simulink subsystem "Propulsion"  (R2023b)
settings: Solver=VariableStepAuto  StartTime=0.0  StopTime=10.0  RelTol=1e-3
undefined symbols (not defined in the file): Thrust, Ts
settings Model: Creator=szdaniel  LastModifiedBy=szdaniel

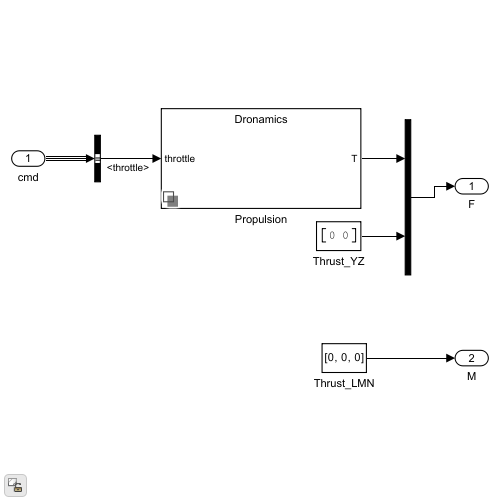
[thumbnail: Simulink's stored preview of the top-level diagram]
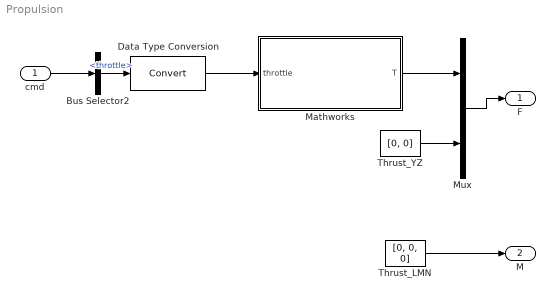
== system Propulsion ==
  cmd : Inport  OutDataTypeStr=Bus: PilotCmdBus  SampleTime=Ts
  Bus Selector2 : BusSelector  OutputSignals=throttle
  Data Type Conversion : DataTypeConversion  SaturateOnIntegerOverflow=off  RndMeth=Floor
  Mathworks : Subsystem  VariantControl=LowFidelityPropulsion
  Mux : Mux  Inputs=[1 2]
  Thrust_LMN : Constant  Value=[0, 0, 0]  SampleTime=Ts
  Thrust_YZ : Constant  Value=[0, 0]  SampleTime=Ts
  F : Outport  Unit=N  VectorParamsAs1DForOutWhenUnconnected=off
  M : Outport  Port=2  Unit=N*m  VectorParamsAs1DForOutWhenUnconnected=off
  wires:
  cmd/1 -> Bus Selector2/1
  Thrust_LMN/1 -> M/1
  Bus Selector2/1 -> Data Type Conversion/1  "<throttle>"
  Mathworks/1(T) -> Mux/1
  Mux/1 -> F/1
  Thrust_YZ/1 -> Mux/2
  Data Type Conversion/1 -> Mathworks/1(throttle)

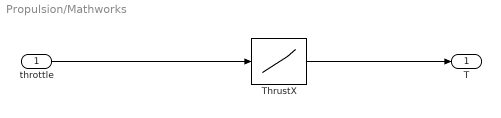
== system Propulsion/Mathworks ==
  throttle : Inport
  ThrustX : Lookup_n-D  NumberOfTableDimensions=1  LookupTableObject=''  BreakpointsForDimension1=(1/6)*(3+([-3:3]))  IndexSearchMethod=Linear search  BeginIndexSearchUsingPreviousIndexResult=on  Table=Thrust*(1+tanh([-3:3]))  ExtrapMethod=Clip
  T : Outport
  wires:
  ThrustX/1 -> T/1
  throttle/1 -> ThrustX/1
